simulink model "lag"  (R2022b)
settings: Solver=VariableStepAuto  StartTime=0.0  StopTime=5000  RelTol=1e-3
undefined symbols (not defined in the file): g1, g3
libraries: simulink x2
settings Model: Creator=amirz  LastModifiedBy=amirz

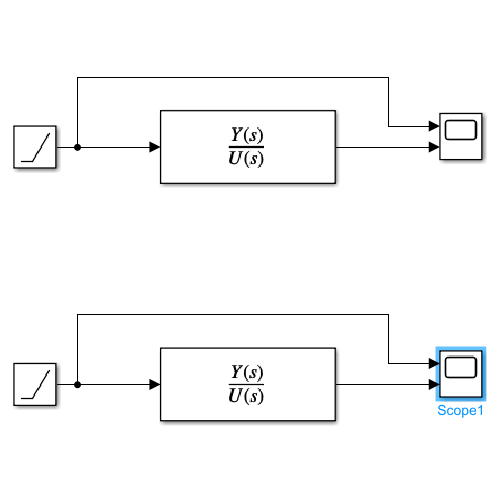
[thumbnail: Simulink's stored preview of the top-level diagram]
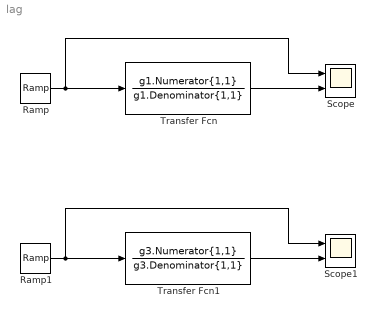
== system lag ==
  Ramp : simulink/Sources/Ramp  slope=1  start=0  InitialOutput=0
  Ramp1 : simulink/Sources/Ramp  slope=1  start=0  InitialOutput=0
  Scope : Scope  NumInputPorts=2
  Scope1 : Scope  NumInputPorts=2
  Transfer Fcn : TransferFcn  Numerator=g1.Numerator{1,1}  Denominator=g1.Denominator{1,1}
  Transfer Fcn1 : TransferFcn  Numerator=g3.Numerator{1,1}  Denominator=g3.Denominator{1,1}
  wires:
  Ramp/1 -> Transfer Fcn/1, Scope/1
  Transfer Fcn/1 -> Scope/2
  Transfer Fcn1/1 -> Scope1/2
  Ramp1/1 -> Transfer Fcn1/1, Scope1/1
